simulink model "ex05_target_fio2_track_object_demo"  (Simulink 7.3)
settings: Solver=FixedStepDiscrete  SolverMode=SingleTasking  StartTime=0.0  StopTime=1  RelTol=1e-3
PreLoadFcn:
  | waijung.modelPreload; % Required for working with Waijung Blockset. Do not remove.
undefined symbols (not defined in the file): A1, A2, A7, B10, B11, B12, C1, C2, C3, C4, C5, Custom, G14, H2, H3, H6, H7, Link, LQFP176, ST, STM32F417IG, system_stm32f4xx
libraries: simulink x11, stm32f4_i2c_lib x8, viptextngfix x2, stm32f4_tim_lib x2, waijung_addon_module x2, waijung_webserver x2, dspsigattribs x1, waijung_image_sensor_lib x1, stm32f4_fsmc_lib x1, stm32f4_rcc_lib x1, stm32f4_device_config_lib x1, waijung_socket_lib x1
(part 1 of 2)
CloseFcn:
  | waijung.modelClose; % Required for working with Waijung Blockset. Do not remove.
settings Model: Creator=Krisada  LastModifiedBy=Krisada
settings OptimizationCC: EnhancedBackFolding=on  OptimizeModelRefInitCode=on  LifeSpan=1
settings HardwareCC: ProdEndianess=LittleEndian  ProdHWDeviceType=ARM Compatible->Cortex - M4  TargetEndianess=LittleEndian  TargetHWDeviceType=ARM Compatible->Cortex - M4
settings RTWCC: SystemTargetFile=stm32f4.tlc  GenerateMakefile=off  TemplateMakefile=ert_default_tmf  Description=STM32F4 Target  ProcessScript=stm32f4_make_rtw_hook
settings CodeAppCC: IgnoreCustomStorageClasses=off
settings STFCustomTargetCC: ModelReferenceCompliant=off  CombineOutputUpdateFcns=on  ERTCustomFileBanners=on  SupportContinuousTime=off  SupportNonInlinedSFcns=off  SystemTargetFile=stm32f4.tlc
settings ERTTargetCC: MultiwordLength=2048  ModelReferenceCompliant=off  ParMdlRefBuildCompliant=off  CompOptLevelCompliant=off  ERTFirstTimeCompliant=off  ModelStepFunctionPrototypeControlCompliant=off  CPPClassGenCompliant=off  ExtModeMexFile=noextcomm  InlinedParameterPlacement=NonHierarchical  ERTSrcFileBannerTemplate=stm32f4_code_template.cgt  ERTHdrFileBannerTemplate=stm32f4_code_template.cgt  ERTDataSrcFileTemplate=stm32f4_code_template.cgt  ERTDataHdrFileTemplate=stm32f4_code_template.cgt  ERTCustomFileTemplate=stm32f4_file_process.tlc

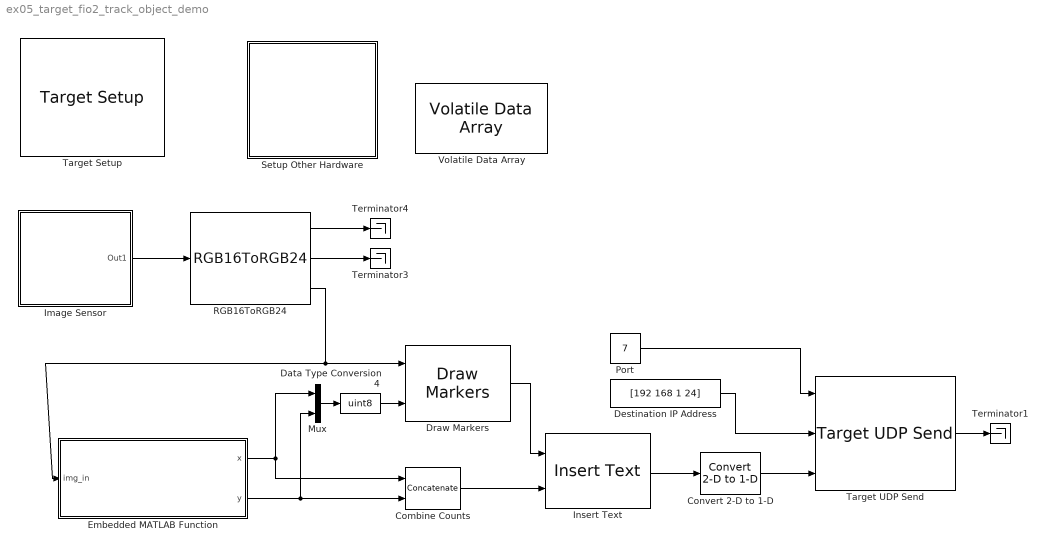
== system ex05_target_fio2_track_object_demo ==
  Combine Counts : Concatenate  Mode=Multidimensional array  ConcatenateDimension=2
  Convert 2-D to 1-D : dspsigattribs/Convert 2-D to 1-D  SystemSampleTime=-1
  Data Type Conversion4 : DataTypeConversion  OutDataTypeMode=uint8  OutDataType=fixdt(1, 16)  OutScaling=2^0  OutDataTypeStr=uint8
  Destination IP Address : Constant  Value=[192 168 1 24]  OutDataTypeMode=uint8  OutDataType=fixdt(1, 16)  OutScaling=2^0  OutDataTypeStr=uint8
  Draw Markers : viptextngfix/Draw Markers  DialogController=vipDDGCreate  DialogControllerArgs=DataTag0  shape=Square  size=5  fill=on  fillClrSource=Specify via dialog  display=White  intensity=200  color=1.5  opacity=0.6  viewport=Entire image  antialiasing=off  inType=Obsolete  imagePorts=One multidimensional signal  prodOutputMode=Binary point scaling  prodOutputWordLength=32  prodOutputFracLength=14  memoryMode=Specify word length  memoryWordLength=16  memoryFracLength=14  roundingMode=Floor  overflowMode=off
  Embedded MATLAB Function : Stateflow chart
  Image Sensor : Subsystem
  Insert Text : viptextngfix/Insert Text  DialogController=vipDDGCreate  DialogControllerArgs=DataTag1  inputType=Obsolete  theText='x: %3.2f, y: %3.2f'  fontFace=LucidaSansRegular  dummyVar1=0  blockFontSize=12  antiAliased=on  getTextLocFrom=Specify via dialog  textLoc=[5 5]  getTextColorFrom=Specify via dialog  textColor=[255 0 0]  getTextIntensityFrom=Specify via dialog  textIntensity=0  getTextOpacityFrom=Specify via dialog  textOpacity=1.0  dummyVar2=0  dummyVar3=0  dummyVar4=0  imagePorts=One multidimensional signal  isInputTransposed=off
  Mux : Mux  Inputs=2
  Port : Constant  Value=7  OutDataTypeMode=uint16  OutDataType=fixdt(1, 16)  OutScaling=2^0  OutDataTypeStr=uint16
  RGB16ToRGB24 : waijung_image_sensor_lib/RGB16ToRGB24  conf=RGB16ToRGB24  column=120  row=160  inputalignment=RGB  outputalignment=BGR  colorseparate=on  simparams=[0 160 0 1]  portpinstr=0  sampletime=-1  blockid=RGB16ToRGB24  inputporttype=[5]  inputportwidth=[19200]  inputportlabel={'Input'}  outputporttype="[3  3 3]"  outputportwidth=[120 120 120]  outputportlabel={'B','G','R'}  compat=0  optionstring="[\"BGR\",\"Param1\"]"
  Setup Other Hardware : Subsystem
  Target Setup : stm32f4_device_config_lib/Target Setup  Priority=100  compiler=GNU ARM  previous_compiler=GNU ARM  mcu=STM32F417IG (LQFP176)  mcustr=STM32F417IG  clockconfig=Custom (system_stm32f4xx.c)  system_stm32f4xx_c_path=F:\trunk\targets\stm32f4_target\stm32f4\utils\STM32F4xx_AN3988_V1.1.0  showmemoryconfiguration=on  stacksize=0x2000  heapsize=0x2000  enableautocompiledownload=on  fullchiperase=off  programmerinterface=ST-Link  editctrlstr=on  compilercontrolstr=$(patsubst %, -I%, .) -mcpu=cortex-m4 -mthumb -mthumb-interwork -mfloat-abi=hard -mfpu=fpv4-sp-d16 -ffast-math -Wall -Wextra -Ofast  assemblercontrolstr=$(patsubst %, -I%, .) -mcpu=cortex-m4 -mthumb -mthumb-interwork -mfloat-abi=hard -mfpu=fpv4-sp-d16 -ffast-math -Wall -Wextra -Ofast -Wa,-amhls=$(<:.s=.lst) -D__STACK_SIZE=$(STACK_SIZE) -D__HEAP_SIZE=$(HEAP_SIZE)  linkercontrolstr=-T$(LD_SCRIPT) -g -Wl,-Map=$(MAP),--cref,--no-warn-mismatch -mcpu=cortex-m4 -mthumb -mthumb-interwork -mfloat-abi=hard -mfpu=fpv4-sp-d16 -specs=nosys.specs  runafterdownload=on  execprofile=None  profileruart=4  profilerbaud=500000  profilertxpin=D8  profilerinitstr=0.01,168000000,1680000,500000,0  manualsetsampletime=off  sampletime=0.01  blockid=TargetSetup  systickreloadvalue=1680000  hseval=8000000  lastprofileruart=4  hclk=168000000  flashorigin=0x8000000  flashlength=1024k  ramorigin=0x64000000  ramlength=0x80000  useextram=on
  Target UDP Send : waijung_socket_lib/Target UDP Send  conf=TargetSend  protocol=UDP  variableipport=on  port=7  address=192.168.1.24  echo=off  transfer=Non-blocking  timeout=5  datasource=VectorStream  streamsource=ExtRAM  streamsize=512  datatype=uint8  datacount=19200  porttype_double=0  porttype_single=0  porttype_int8=0  porttype_uint8=0  porttype_int16=0  porttype_uint16=0  porttype_int32=0  porttype_uint32=1  portpinstr=0  sampletime=-1  blockid=TargetUDPSend  inputporttype=[5,3,3]  inputportwidth=[1,4,19200]  inputportlabel={'Port','IP','Data(1:19200)'}  outputporttype=[7]  outputportwidth=[]  outputportlabel={'Status'}  compat=0  optionstring="[\"UDP\",\"7\",\"192\",\"168\",\"1\",\"24\",\"Non-blocking\",\"VectorStream\",\"uint8_t\",\"19200\",\"Send\",\"off\",\"on\",\"\",\"\",\"\",\"\",\"\",\"512\"]"  options=[7,2,0,5000,0]
  Terminator1 : Terminator
  Terminator3 : Terminator
  Terminator4 : Terminator
  Volatile Data Array : waijung_addon_module/Data Storage/Volatile Data Array  conf=Setup  specificaddress=off  storagename=ExtRAM  memoryaddress=hex2dec('64000000')  storagetype=uint16  datasize=160*120  varname=VolatileDataArray_ExtRAM  datatype=double  datacount=0  portpinstr=0  sampletime=inf  blockid=VolatileDataArray  inputporttype=[]  inputportwidth=[]  inputportlabel={}  outputporttype=[]  outputportwidth=[]  outputportlabel={}  compat=0  optionstring="[\"off\",\"?\",\"ExtRAM\",\"uint16\",\"19200\",\"VolatileDataArray_ExtRAM\",\"uint16_t\",\"Param1\"]"
  wires:
  Image Sensor/1(Out1) -> RGB16ToRGB24/1
  RGB16ToRGB24/2 -> Terminator3/1
  RGB16ToRGB24/1 -> Terminator4/1
  Mux/1 -> Data Type Conversion4/1
  Data Type Conversion4/1 -> Draw Markers/2
  Draw Markers/1 -> Insert Text/1
  Combine Counts/1 -> Insert Text/2
  Embedded MATLAB Function/1(x) -> Mux/1, Combine Counts/1
  Embedded MATLAB Function/2(y) -> Mux/2, Combine Counts/2
  Insert Text/1 -> Convert 2-D to 1-D/1
  Destination IP Address/1 -> Target UDP Send/2
  Port/1 -> Target UDP Send/1
  Target UDP Send/1 -> Terminator1/1
  Convert 2-D to 1-D/1 -> Target UDP Send/3
  RGB16ToRGB24/3 -> Embedded MATLAB Function/1(img_in), Draw Markers/1

== system ex05_target_fio2_track_object_demo/Image Sensor ==
  Camera OV1 : Subsystem  mask{camera=OV7670, storagename=ExtRAM, xclkfreq=8MHz(MCO), imgsize=120 x 160, module=1, slvaddr=hex2dec('42'), sampletime=0.1}
      mask prompts: storagename "Output buffer"; xclkfreq "XCLK input frequency"; imgsize "Image size"; module "I2C Module"; slvaddr "I2C Slave address"; sampletime "Sample time (sec)"
      mask init:
      | waijung_image_sensor_callback('init');
      mask StyleString: popup(OV7670),popup(ExtRAM|ExtRAM),popup(8MHz(MCO)|24MHz),popup(120 x 160|240 x 320|480 x 640),popup(1|2|3),edit,edit
      mask CallbackString: waijung_image_sensor_callback('camera');|waijung_image_sensor_callback('storagename');|||waijung_image_sensor_callback('module');||
      mask Display: text(0.5, 0.5, '[OV7670]\nPort: I2C1','ver','middle','hor','center');port_label('output', 1,'READY');
  Constant2 : Constant  Value=0  OutDataTypeMode=uint32  OutDataType=fixdt(1, 16)  OutScaling=2^0  OutDataTypeStr=uint32  SampleTime=0.1
  Terminator : Terminator
  Volatile Data Array Read : waijung_addon_module/Data Storage/Volatile Data Array Read  conf=Read  specificaddress=off  storagename=ExtRAM  memoryaddress=hex2dec('64000000')  storagetype=uint8  datasize=120*160*3  varname=VolatileDataArray_ExtRAM  datatype=uint8  datacount=128  variablesize=off  portpinstr=0  sampletime=inf  blockid=ImageSensorVolatileDataArrayRead  inputporttype=[7]  inputportwidth=[1]  inputportlabel={'Offset'}  outputporttype=[3]  outputportwidth=[128]  outputportlabel={'Data(128)'}  compat=0  optionstring="[\"ExtRAM\",\"uint16\",\"19200\",\"VolatileDataArray_ExtRAM\",\"uint16_t\",\"uint16\",\"uint16_t\",\"19200\",\"Param1\"]"
  Out1 : Outport
  wires:
  Constant2/1 -> Volatile Data Array Read/1
  Camera OV1/1(Data) -> Terminator/1
  Volatile Data Array Read/1 -> Out1/1

== system ex05_target_fio2_track_object_demo/Setup Other Hardware ==
  Ethernet Application Setup : waijung_webserver/Ethernet Application Setup  conf=Setup  ipaddress=192.168.1.31  netmask=255.255.255.0  gateway=192.168.1.1  macaddress=02-00-00-00-00-00  dhcp=off  timerscaler=100  portpinstr=0  sampletime=0.0001  blockid=SetupOtherHardwareEthernetApplicationSetup  inputporttype=[]  inputportwidth=[]  inputportlabel={}  outputporttype=[]  outputportwidth=[]  outputportlabel={}  compat=0  optionstring="[\"Dummy\",\"192\",\"168\",\"1\",\"31\",\"255\",\"255\",\"255\",\"0\",\"192\",\"168\",\"1\",\"1\",\"02\",\"00\",\"00\",\"00\",\"00\",\"00\",\"off\",\"100\"]"
  Ethernet Link Setup1 : waijung_webserver/Ethernet Link Setup  conf=Setup  interfacepin=Profile #2  wj_interfacetype=MII  pin_mdio=A2  pin_mdc=C1  pin_pps=Not used  pin_crs=H2  pin_col=H3  pin_dv=A7  pin_rxclk=A1  pin_rxer=B10  pin_rxd0=C4  pin_rxd1=C5  pin_rxd2=H6  pin_rxd3=H7  pin_txclk=C3  pin_txen=B11  pin_txd0=B12  pin_txd1=G14  pin_txd2=C2  pin_txd3=E2  portpinstr=H2,A1,A2,H3,A7,H6,H7,E2,B10,B11,B12,G14,C1,C2,C3,C4,C5  sampletime=inf  blockid=SetupOtherHardwareEthernetLinkSetup1  inputporttype=[]  inputportwidth=[]  inputportlabel={}  outputporttype=[]  outputportwidth=[]  outputportlabel={}  compat=0  optionstring="[\"xxx\",\"on\",\"on\",\"on\",\"off\",\"on\",\"off\",\"on\",\"on\",\"off\",\"on\",\"on\",\"on\",\"on\",\"on\",\"on\",\"on\",\"off\",\"on\",\"on\",\"on\",\"on\",\"on\",\"on\",\"on\",\"on\",\"on\",\"on\",\"H\",\"2\",\"A\",\"1\",\"A\",\"2\",\"H\",\"3\",\"A\",\"7\",\"H\",\"6\",\"H\",\"7\",\"N\",\"ot used\",\"E\",\"2\",\"B\",\"10\",\"B\",\"11\",\"B\",\"12\",\"G\",\"14\",\"C\",\"1\",\"C\",\"2\",\"C\",\"3\",\"C\",\"4\",\"C\",\"5\",\"MII\"]"
  FSMC_SRAM Setup : stm32f4_fsmc_lib/FSMC_SRAM Setup  conf=RamSetup  useextmem=on  extmemaddress=hex2dec('64000000')  extramsize=hex2dec('80000')  datasource=0x64000000  sampletime=inf  sampletimestr=0  blockid=SetupOtherHardwareFSMC_SRAMSetup  inputarray=[]  inputlabelarray={}  outputarray=[]  outputlabelarray={}  compat=0  confstr="[\"on\"]"
  I2C Master Setup : S-Function  FunctionName=stm32f4_i2c  Parameters=configuration,module,transfer,clkspeed,timeout,sdapin,sclpin,writecount,readcount,inputtypearray,outputtypearray,confstr,sampletime,sampletimestr,blockid  EnableBusSupport=off  mask(stm32f4_i2c){configuration=Setup, module=1, lastmodule=1, transfer=Blocking, dutycycle=TLow/THigh = 2, clkspeed=100, timeout=25, writecount=0, readcount=0, sdapin=B7, sclpin=B6, waitwritetime=0, inputtypearray=[0], outputtypearray=[0], confstr=["B","7","B","6","1","1","6","0","I2C_DutyCycle_2","0","off"], sampletime=-1, sampletimestr=0, blockid=SetupOtherHardwareI2CMasterSetup}
      mask prompts: module "I2C Module"; lastmodule "Last module"; transfer "Transfer mode"; dutycycle "Duty cycle in fast mode"; clkspeed "Clock speed (kHz)"; timeout "Timeout (ms)"; writecount "Bytes write count"; readcount "Bytes read count"; sdapin "SDA pin"; sclpin "SCL pin"; waitwritetime "Wait write time (ms), default is 0"; inputtypearray "Input type array"; outputtypearray "Output type array"; confstr "Configuration string"; sampletime "Sample time (sec)"; sampletimestr "Compiled sample time (sec) in string"
      mask init:
      | stm32f4_i2c_callback('init');
      mask Help: web(fullfile(waijungdocroot,'stm32f4_i2c_setup.htm'), '-browser')
      mask StyleString: popup(Setup|Transaction),popup(1|2|3),edit,popup(Blocking|Non-blocking),popup(TLow/THigh = 16/9|TLow/THigh = 2),edit,edit,edit,edit,popup(Not used|B7|B9),popup(Not used|B6|B8),edit,edit,edit,edit,edit,edit,edit
      mask CallbackString: stm32f4_i2c_callback('configuration');|stm32f4_i2c_callback('module');|||stm32f4_i2c_callback('dutycycle');|||stm32f4_i2c_callback('writecount');|stm32f4_i2c_callback('readcount');|stm32f4_i2c_callback('sdapin');|stm32f4_i2c_callback('sclpin');||||stm32f4_i2c_callback('confstr');|stm32f4_i2c_callback('sampletime');|stm32f4_i2c_callback('sampletimestr');|stm32f4_i2c_callback('blockid');
      mask Display: text(0.5, 0.5, 'Module: I2C1\nClock: 100kHz\nSDA/SCL Pin: B7/B6','ver','middle','hor','center');
  MCO : stm32f4_rcc_lib/MCO  conf=MCO  module=1  source=HSE  div=Div_1  sampletime=inf  sampletimestr=0  blockid=SetupOtherHardwareMCO  inputarray=[]  inputlabelarray={}  outputarray=[]  outputlabelarray={}  compat=0  confstr="[\"1\",\"HSE\",\"Div_1\"]"

== system ex05_target_fio2_track_object_demo/Image Sensor/Camera OV1 ==
  Capture_ : Subsystem  TreatAsAtomicUnit=on
  Init_ : Subsystem
  Logical Operator : Logic  Operator=NOT  AllPortsSameDT=off  OutDataTypeMode=boolean  LogicDataType=fixdt(0, 8)  OutDataTypeStr=boolean
  Memory : Memory  InheritSampleTime=on
  Rate Transition : RateTransition  OutPortSampleTime=sampletime
  Data : Outport  OutDataType=fixdt(1, 16)  OutScaling=2^0
  wires:
  Rate Transition/1 -> Capture_/Enable
  Logical Operator/1 -> Init_/Enable
  Memory/1 -> Rate Transition/1, Logical Operator/1
  Init_/1(Out1) -> Memory/1
  Capture_/1(SUCCESS) -> Data/1

== system ex05_target_fio2_track_object_demo/Image Sensor/Camera OV1/Capture_ ==
  Enable : EnablePort
  Compare To Zero : simulink/Logic and Bit Operations/Compare To Zero  SystemSampleTime=-1  relop===  LogicOutDataTypeMode=uint8  ZeroCross=off
  DCMI Capture : S-Function  FunctionName=stm32f4_dcmi  Parameters=conf,inputporttype,inputportwidth,outputporttype,outputportwidth,optionstring,sampletime,blockid  EnableBusSupport=off  mask(stm32f4_dcmi){conf=DCMI, capturemode=SnapShot, synchronizemode=Hardware, pclkpolarity=Falling, vspolarity=High, hspolarity=High, capturerate=All, capturesize=120*160*2, storagename=<Manual Configure>, varname=VolatileDataArray_ExtRAM, storagetype=uint16, storagesize=120*160, remap=Profile #2, sampletime=inf, blockid=ImageSensorCameraOV1Capture_DCMICapture, inputporttype=[], inputportwidth=[], inputportlabel={}, outputporttype=[7], outputportwidth=[], outputportlabel={'Status'}, compat=0, optionstring=["DCMI","SnapShot","Hardware","Falling","High","High","All","0","HalfWord","9600","0","0","VolatileDataArray_ExtRAM"," "," "," ","1","0","0","0","0","0","0","1","1","A","6","I","5","H","8","H","9","H","10","H","11","H","12","H","14","I","4","I","6","I","7"], portpinstr=A6,I5,H8,H9,H10,H11,H12,H14,I4,I6,I7}
      mask prompts: conf "Configuration"; capturemode "Capture mode"; synchronizemode "Synchronization Mode"; pclkpolarity "Pixel clock polarity"; vspolarity "Vertical synchronization polarity"; hspolarity "Horizontal synchronization polarity"; capturerate "Capture rate"; capturesize "Capture data size (Bytes)"; storagename "Output buffer"; varname "Output buffer var name"; storagetype "Output buffer var type"; storagesize "Output buffer size (Total bytes must be equal to, or greater than DMA Transfer size)"; remap "Remap DCMI pins"; sampletime "Sample time (sec)"; inputporttype "Input port"; inputportwidth "Input Port Width"; inputportlabel "Input port label"; outputporttype "Output port"; outputportwidth "Output Port Width"; outputportlabel "Output port label"; compat "Compatibility (Reserved for future use)"; optionstring "Configuration String"; portpinstr "Port Pin String"
      mask help:
      | Synchronize mode:
      |  - Hardware: Hardware synchronization data capture is synchronized with the HSYNC/VSYNC signals.
      |  - Embedded: Embedded synchronization data capture is synchronized with synchronization codes embedded in the data flow.
      | Pixel clock polarity:
      |  - Falling: Pixel clock active on Falling edge.
      |  - Rising: Pixel clock active on Rising edge.
      | Vertical, Horizontal sychronization polarity:
      |  - Low: vertical synchronization active Low.
      |  - High: Vertical synchronization active High.
      | Capture rate:
      |  - All: All frames are captured.
      |  - 1of2: Every alternate frame captured.
      |  - 1of4: On frame in 4 frames captured.
      | Pins Profile:
      | Set of configuration pins for: PIXCLK, VSYNC, HSYNC, D0, D1, .., D7 corresponding.
      |  - Profile #1: PA6, PB7, PA4, PC6, PC7,  PE0,  PE1,  PE4,  PB6, PE5, PE6
      |  - Profile #2: PA6, PI5, PH8, PH9, PH10, PH11, PH12, PH14, PI4, PI6, PI7
      mask init:
      | stm32f4_dcmi_callback('init');
      mask Help: web(fullfile(waijungdocroot,'stm32f4_dcmi.htm'), '-browser')
      mask StyleString: popup(DCMI),popup(Continuous|SnapShot),popup(Hardware|Embedded),popup(Falling|Rising),popup(High|Low),popup(High|Low),popup(All|1of2|1of4),edit,popup(<Manual Configure>),edit,popup(double|single|int8|uint8|int16|uint16|int32|uint32),edit,popup(Profile #1|Profile #2),edit,edit,edit,edit,edit,edit,edit,edit,edit,edit,edit
      mask CallbackString: stm32f4_dcmi_callback('conf');||||||||stm32f4_dcmi_callback('storagename');|||stm32f4_dcmi_callback('storagesize');|stm32f4_dcmi_callback('remap');|stm32f4_dcmi_callback('sampletime');|stm32f4_dcmi_callback('blockid');|||||||||
      mask Display: text(0.05, 0.5, 'Size: 38400\nPins: Profile #2\nTs (sec): 0','ver','middle','hor','left'); port_label('output', 1,'Status');
  SUCCESS : Outport  OutDataType=fixdt(1, 16)  OutScaling=2^0
  wires:
  DCMI Capture/1 -> Compare To Zero/1
  Compare To Zero/1 -> SUCCESS/1

== system ex05_target_fio2_track_object_demo/Image Sensor/Camera OV1/Init_ ==
  Enable : EnablePort
  While Iterator_ : Subsystem  TreatAsAtomicUnit=on
  Out1 : Outport
  wires:
  While Iterator_/1(Ready) -> Out1/1

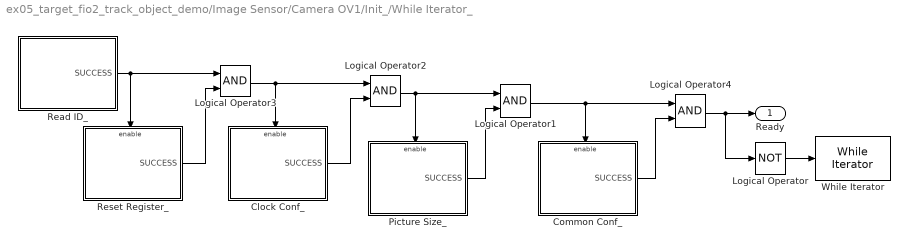
== system ex05_target_fio2_track_object_demo/Image Sensor/Camera OV1/Init_/While Iterator_ ==
  Clock Conf_ : Subsystem
  Common Conf_ : Subsystem
  Logical Operator : Logic  Operator=NOT  AllPortsSameDT=off  OutDataTypeMode=boolean  LogicDataType=fixdt(0, 8)  OutDataTypeStr=boolean
  Logical Operator{1..4} (4 alike) : Logic  AllPortsSameDT=off  OutDataTypeMode=boolean  LogicDataType=fixdt(0, 8)  OutDataTypeStr=boolean
  Picture Size_ : Subsystem
  Read ID_ : Subsystem
  Reset Register_ : Subsystem
  While Iterator : WhileIterator  MaxIters=-1  WhileBlockType=do-while
  Ready : Outport  OutDataType=fixdt(1, 16)  OutScaling=2^0
  wires:
  Common Conf_/1(SUCCESS) -> Logical Operator4/2
  Logical Operator4/1 -> Ready/1, Logical Operator/1
  Logical Operator2/1 -> Picture Size_/Enable, Logical Operator1/1
  Clock Conf_/1(SUCCESS) -> Logical Operator2/2
  Reset Register_/1(SUCCESS) -> Logical Operator3/2
  Logical Operator/1 -> While Iterator/1
  Logical Operator1/1 -> Logical Operator4/1, Common Conf_/Enable
  Picture Size_/1(SUCCESS) -> Logical Operator1/2
  Read ID_/1(SUCCESS) -> Logical Operator3/1, Reset Register_/Enable
  Logical Operator3/1 -> Logical Operator2/1, Clock Conf_/Enable

== system ex05_target_fio2_track_object_demo/Image Sensor/Camera OV1/Init_/While Iterator_/Clock Conf_ ==
  Enable : EnablePort
  Logical Operator : Logic  Operator=NOT  AllPortsSameDT=off  OutDataTypeMode=boolean  LogicDataType=fixdt(0, 8)  OutDataTypeStr=boolean
  Memory : Memory  InheritSampleTime=on
  Subsystem : Subsystem
  SUCCESS : Outport  OutDataType=fixdt(1, 16)  OutScaling=2^0
  wires:
  Subsystem/1(Out1) -> SUCCESS/1, Memory/1
  Logical Operator/1 -> Subsystem/Enable
  Memory/1 -> Logical Operator/1

== system ex05_target_fio2_track_object_demo/Image Sensor/Camera OV1/Init_/While Iterator_/Common Conf_ ==
  Enable : EnablePort
  Logical Operator : Logic  Operator=NOT  AllPortsSameDT=off  OutDataTypeMode=boolean  LogicDataType=fixdt(0, 8)  OutDataTypeStr=boolean
  Memory : Memory  InheritSampleTime=on
  Subsystem : Subsystem
  SUCCESS : Outport  OutDataType=fixdt(1, 16)  OutScaling=2^0
  wires:
  Subsystem/1(Out1) -> SUCCESS/1, Memory/1
  Logical Operator/1 -> Subsystem/Enable
  Memory/1 -> Logical Operator/1

== system ex05_target_fio2_track_object_demo/Image Sensor/Camera OV1/Init_/While Iterator_/Picture Size_ ==
  Enable : EnablePort
  Logical Operator : Logic  Operator=NOT  AllPortsSameDT=off  OutDataTypeMode=boolean  LogicDataType=fixdt(0, 8)  OutDataTypeStr=boolean
  Memory : Memory  InheritSampleTime=on
  Subsystem : Subsystem
  SUCCESS : Outport  OutDataType=fixdt(1, 16)  OutScaling=2^0
  wires:
  Memory/1 -> Logical Operator/1
  Logical Operator/1 -> Subsystem/Enable
  Subsystem/1(Out1) -> Memory/1, SUCCESS/1

== system ex05_target_fio2_track_object_demo/Image Sensor/Camera OV1/Init_/While Iterator_/Read ID_ ==
  Logical Operator : Logic  Operator=NOT  AllPortsSameDT=off  OutDataTypeMode=boolean  LogicDataType=fixdt(0, 8)  OutDataTypeStr=boolean
  Memory : Memory  InheritSampleTime=on
  Subsystem_ : Subsystem
  SUCCESS : Outport  OutDataType=fixdt(1, 16)  OutScaling=2^0
  wires:
  Memory/1 -> Logical Operator/1
  Logical Operator/1 -> Subsystem_/Enable
  Subsystem_/1(Out1) -> Memory/1, SUCCESS/1

== system ex05_target_fio2_track_object_demo/Image Sensor/Camera OV1/Init_/While Iterator_/Reset Register_ ==
  Enable : EnablePort
  Logical Operator : Logic  Operator=NOT  AllPortsSameDT=off  OutDataTypeMode=boolean  LogicDataType=fixdt(0, 8)  OutDataTypeStr=boolean
  Memory : Memory  InheritSampleTime=on
  Subsystem : Subsystem
  SUCCESS : Outport  OutDataType=fixdt(1, 16)  OutScaling=2^0
  wires:
  Subsystem/1(Out1) -> SUCCESS/1, Memory/1
  Logical Operator/1 -> Subsystem/Enable
  Memory/1 -> Logical Operator/1

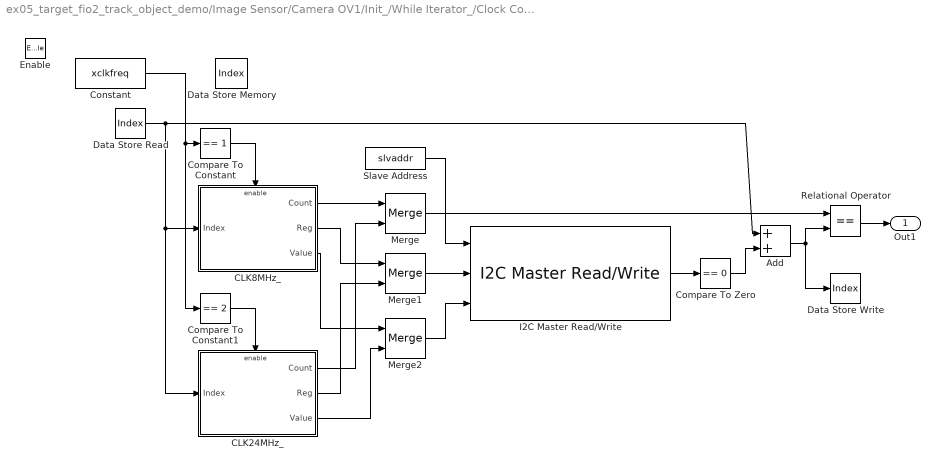
== system ex05_target_fio2_track_object_demo/Image Sensor/Camera OV1/Init_/While Iterator_/Clock Conf_/Subsystem ==
  Enable : EnablePort
  Add : Sum  OutDataType=fixdt(1, 16)  OutScaling=2^-10
  CLK24MHz_ : Subsystem  TreatAsAtomicUnit=on
  CLK8MHz_ : Subsystem  TreatAsAtomicUnit=on
  Compare To Constant : simulink/Logic and Bit Operations/Compare To Constant  SystemSampleTime=-1  relop===  const=1  LogicOutDataTypeMode=boolean  ZeroCross=off
  Compare To Constant1 : simulink/Logic and Bit Operations/Compare To Constant  SystemSampleTime=-1  relop===  const=2  LogicOutDataTypeMode=boolean  ZeroCross=off
  Compare To Zero : simulink/Logic and Bit Operations/Compare To Zero  SystemSampleTime=-1  relop===  LogicOutDataTypeMode=uint8  ZeroCross=off
  Constant : Constant  Value=xclkfreq  OutDataType=fixdt(1, 16)  OutScaling=2^0
  Data Store Memory : DataStoreMemory  DataStoreName=Index  ReadBeforeWriteMsg=warning  WriteAfterWriteMsg=warning  WriteAfterReadMsg=warning  DataType=uint8  OutDataType=fixdt(1, 16)  OutScaling=2^0  OutDataTypeStr=uint8
  Data Store Read : DataStoreRead  DataStoreName=Index  SampleTime=-1
  Data Store Write : DataStoreWrite  DataStoreName=Index  SampleTime=-1
  I2C Master Read/Write : stm32f4_i2c_lib/I2C Master Read//Write  configuration=Transaction  module=1  lastmodule=3  transfer=Blocking  dutycycle=TLow/THigh = 2  clkspeed=400  timeout=25  writecount=2  readcount=0  sdapin=C9  sclpin=A8  waitwritetime=5  forcestop=off  inputtypearray=[3 3 3 3]  outputtypearray=[1 3]  confstr="[\"C\",\"9\",\"A\",\"8\",\"1\",\"1\",\"6\",\"0\",\"I2C_DutyCycle_2\",\"5\",\"off\"]"  sampletime=-1  sampletimestr=0  blockid=ImageSensorCameraOV1Init_WhileIterator_ClockConf_SubsystemI2CMasterReadWrite
  Merge : Merge
  Merge1 : Merge
  Merge2 : Merge
  Relational Operator : RelationalOperator  Operator===  LogicOutDataTypeMode=boolean  LogicDataType=fixdt(0, 8)  OutDataTypeStr=boolean
  Slave Address : Constant  Value=slvaddr  OutDataTypeMode=uint8  OutDataType=fixdt(1, 16)  OutScaling=2^0  OutDataTypeStr=uint8
  Out1 : Outport
  wires:
  Merge2/1 -> I2C Master Read/Write/3
  Merge1/1 -> I2C Master Read/Write/2
  Merge/1 -> Relational Operator/1
  Constant/1 -> Compare To Constant1/1, Compare To Constant/1
  CLK24MHz_/3(Value) -> Merge2/2
  CLK24MHz_/2(Reg) -> Merge1/2
  CLK24MHz_/1(Count) -> Merge/2
  CLK8MHz_/3(Value) -> Merge2/1
  CLK8MHz_/2(Reg) -> Merge1/1
  CLK8MHz_/1(Count) -> Merge/1
  Compare To Constant1/1 -> CLK24MHz_/Enable
  Compare To Constant/1 -> CLK8MHz_/Enable
  Slave Address/1 -> I2C Master Read/Write/1
  Data Store Read/1 -> CLK24MHz_/1(Index), CLK8MHz_/1(Index), Add/1
  I2C Master Read/Write/1 -> Compare To Zero/1
  Compare To Zero/1 -> Add/2
  Add/1 -> Relational Operator/2, Data Store Write/1
  Relational Operator/1 -> Out1/1

== system ex05_target_fio2_track_object_demo/Image Sensor/Camera OV1/Init_/While Iterator_/Common Conf_/Subsystem ==
  Enable : EnablePort
  Add : Sum  OutDataType=fixdt(1, 16)  OutScaling=2^-10
  Compare To Zero : simulink/Logic and Bit Operations/Compare To Zero  SystemSampleTime=-1  relop===  LogicOutDataTypeMode=uint8  ZeroCross=off
  Data Store Memory : DataStoreMemory  DataStoreName=Index  ReadBeforeWriteMsg=warning  WriteAfterWriteMsg=warning  WriteAfterReadMsg=warning  DataType=uint8  OutDataType=fixdt(1, 16)  OutScaling=2^0  OutDataTypeStr=uint8
  Data Store Read : DataStoreRead  DataStoreName=Index  SampleTime=-1
  Data Store Write : DataStoreWrite  DataStoreName=Index  SampleTime=-1
  I2C Master Read/Write : stm32f4_i2c_lib/I2C Master Read//Write  configuration=Transaction  module=1  lastmodule=3  transfer=Blocking  dutycycle=TLow/THigh = 2  clkspeed=400  timeout=25  writecount=2  readcount=0  sdapin=C9  sclpin=A8  waitwritetime=5  forcestop=off  inputtypearray=[3 3 3 3]  outputtypearray=[1 3]  confstr="[\"C\",\"9\",\"A\",\"8\",\"1\",\"1\",\"6\",\"0\",\"I2C_DutyCycle_2\",\"5\",\"off\"]"  sampletime=-1  sampletimestr=0  blockid=ImageSensorCameraOV1Init_WhileIterator_CommonConf_SubsystemI2CMasterReadWrite
  Register List : Subsystem  mask{register=uint8([122,123,124,125,126,127,128,129,130,131,132,133,134,135,136,137,19,21,0,16,13,20,165,171,36,37,38,159,160,161,166,167,168,169,170,19,14,15,22,30,33,34,41,51,53,55,56,57,60,77,78,105,116,141,142,143,144,145,146,150,154,176,177,178,179,184,67,68,69,70,71,72,89,90,91,92,93,94,100,101,102,148,149,108,109,110,111,106,1,2,19,21,79,80,81,82,83,84,85,86,87,88,65,63,117,118,76,119,75,201,65,86,52,59,164,150,157,158,9,59]), value=uint8([32,28,40,60,85,104,118,128,136,143,150,163,175,196,215,232,232,24,15,0,0,32,5,7,117,99,165,120,104,3,223,223,240,144,148,229,97,75,2,39,2,145,7,11,11,29,113,42,120,64,32,0,25,79,0,0,0,0,0,0,128,132,12,14,130,10,20,240,52,88,40,58,136,136,68,103,73,14,4,32,5,4,8,10,85,17,159,64,64,64,231,24,128,128,0,34,94,128,0,82,128,158,8,5,5,225,15,10,9,192,56,64,17,2,137,0,76,63,2,66])}
      mask prompts: register "Register Index"; value "Register Value"
      mask help:
      | Count:
      |  - Number of Register-Value pair.
      |  - Determine from lowest size, between Register and Value.
      | Reg:
      |  - Register index.
      | Value:
      |  - Data corresponding to specified register index.
  Relational Operator : RelationalOperator  Operator===  LogicOutDataTypeMode=boolean  LogicDataType=fixdt(0, 8)  OutDataTypeStr=boolean
  Slave Address : Constant  Value=slvaddr  OutDataTypeMode=uint8  OutDataType=fixdt(1, 16)  OutScaling=2^0  OutDataTypeStr=uint8
  Out1 : Outport
  wires:
  Slave Address/1 -> I2C Master Read/Write/1
  Data Store Read/1 -> Add/1, Register List/1(Index)
  I2C Master Read/Write/1 -> Compare To Zero/1
  Compare To Zero/1 -> Add/2
  Add/1 -> Relational Operator/2, Data Store Write/1
  Relational Operator/1 -> Out1/1
  Register List/2(Reg) -> I2C Master Read/Write/2
  Register List/3(Value) -> I2C Master Read/Write/3
  Register List/1(Count) -> Relational Operator/1

== system ex05_target_fio2_track_object_demo/Image Sensor/Camera OV1/Init_/While Iterator_/Picture Size_/Subsystem ==
  Enable : EnablePort
  Add : Sum  OutDataType=fixdt(1, 16)  OutScaling=2^-10
  Compare To Zero : simulink/Logic and Bit Operations/Compare To Zero  SystemSampleTime=-1  relop===  LogicOutDataTypeMode=uint8  ZeroCross=off
  Data Store Memory : DataStoreMemory  DataStoreName=Index  ReadBeforeWriteMsg=warning  WriteAfterWriteMsg=warning  WriteAfterReadMsg=warning  DataType=uint8  OutDataType=fixdt(1, 16)  OutScaling=2^0  OutDataTypeStr=uint8
  Data Store Read : DataStoreRead  DataStoreName=Index  SampleTime=-1
  Data Store Write : DataStoreWrite  DataStoreName=Index  SampleTime=-1
  I2C Master Read/Write : stm32f4_i2c_lib/I2C Master Read//Write  configuration=Transaction  module=1  lastmodule=3  transfer=Blocking  dutycycle=TLow/THigh = 2  clkspeed=400  timeout=25  writecount=2  readcount=0  sdapin=C9  sclpin=A8  waitwritetime=5  forcestop=off  inputtypearray=[3 3 3 3]  outputtypearray=[1 3]  confstr="[\"C\",\"9\",\"A\",\"8\",\"1\",\"1\",\"6\",\"0\",\"I2C_DutyCycle_2\",\"5\",\"off\"]"  sampletime=-1  sampletimestr=0  blockid=ImageSensorCameraOV1Init_WhileIterator_PictureSize_SubsystemI2CMasterReadWrite
  Relational Operator : RelationalOperator  Operator===  LogicOutDataTypeMode=boolean  LogicDataType=fixdt(0, 8)  OutDataTypeStr=boolean
  Slave Address : Constant  Value=slvaddr  OutDataTypeMode=uint8  OutDataType=fixdt(1, 16)  OutScaling=2^0  OutDataTypeStr=uint8
  Subsystem : Subsystem
  Out1 : Outport
  wires:
  Subsystem/1(Count) -> Relational Operator/1
  Subsystem/2(Reg) -> I2C Master Read/Write/2
  Subsystem/3(Value) -> I2C Master Read/Write/3
  Relational Operator/1 -> Out1/1
  Add/1 -> Data Store Write/1, Relational Operator/2
  Compare To Zero/1 -> Add/2
  I2C Master Read/Write/1 -> Compare To Zero/1
  Data Store Read/1 -> Subsystem/1(Index), Add/1
  Slave Address/1 -> I2C Master Read/Write/1

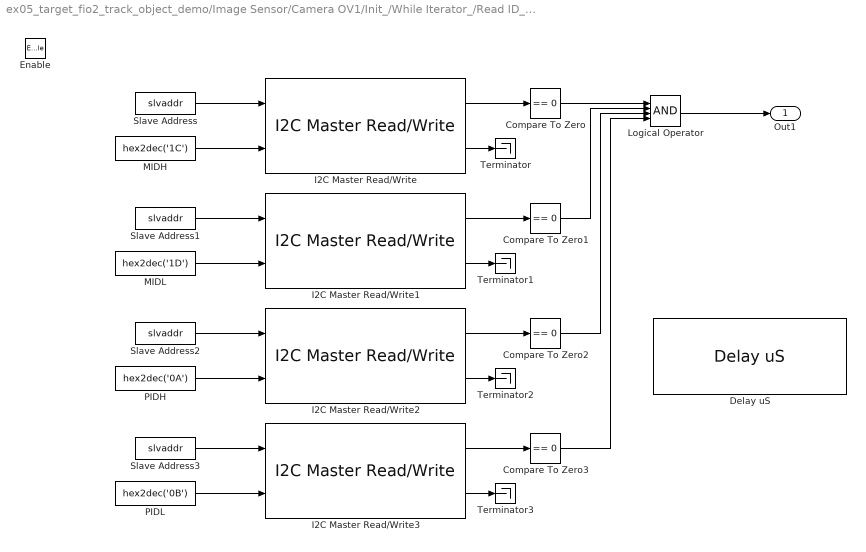
== system ex05_target_fio2_track_object_demo/Image Sensor/Camera OV1/Init_/While Iterator_/Read ID_/Subsystem_ ==
  Enable : EnablePort
  Compare To Zero{,1..3} (4 alike) : simulink/Logic and Bit Operations/Compare To Zero  SystemSampleTime=-1  relop===  LogicOutDataTypeMode=uint8  ZeroCross=off
  Delay uS : stm32f4_tim_lib/Delay uS  Priority=0  delaytime=300000  enableinput=off  enableoutput=off  inputtypearray=[0]  outputtypearray=[0]  sampletime=-1  sampletimestr=0  blockid=ImageSensorCameraOV1Init_WhileIterator_ReadID_Subsystem_DelayuS
  I2C Master Read/Write : stm32f4_i2c_lib/I2C Master Read//Write  configuration=Transaction  module=1  lastmodule=3  transfer=Blocking  dutycycle=TLow/THigh = 2  clkspeed=400  timeout=25  writecount=1  readcount=1  sdapin=C9  sclpin=A8  waitwritetime=0  forcestop=on  inputtypearray=[2 3 3]  outputtypearray=[2 3 3]  confstr="[\"C\",\"9\",\"A\",\"8\",\"1\",\"1\",\"6\",\"0\",\"I2C_DutyCycle_2\",\"0\",\"on\"]"  sampletime=-1  sampletimestr=0  blockid=ImageSensorCameraOV1Init_WhileIterator_ReadID_Subsystem_I2CMasterReadWrite
  I2C Master Read/Write1 : stm32f4_i2c_lib/I2C Master Read//Write  configuration=Transaction  module=1  lastmodule=3  transfer=Blocking  dutycycle=TLow/THigh = 2  clkspeed=400  timeout=25  writecount=1  readcount=1  sdapin=C9  sclpin=A8  waitwritetime=0  forcestop=on  inputtypearray=[2 3 3]  outputtypearray=[2 3 3]  confstr="[\"C\",\"9\",\"A\",\"8\",\"1\",\"1\",\"6\",\"0\",\"I2C_DutyCycle_2\",\"0\",\"on\"]"  sampletime=-1  sampletimestr=0  blockid=ImageSensorCameraOV1Init_WhileIterator_ReadID_Subsystem_I2CMasterReadWrite1
  I2C Master Read/Write2 : stm32f4_i2c_lib/I2C Master Read//Write  configuration=Transaction  module=1  lastmodule=3  transfer=Blocking  dutycycle=TLow/THigh = 2  clkspeed=400  timeout=25  writecount=1  readcount=1  sdapin=C9  sclpin=A8  waitwritetime=0  forcestop=on  inputtypearray=[2 3 3]  outputtypearray=[2 3 3]  confstr="[\"C\",\"9\",\"A\",\"8\",\"1\",\"1\",\"6\",\"0\",\"I2C_DutyCycle_2\",\"0\",\"on\"]"  sampletime=-1  sampletimestr=0  blockid=ImageSensorCameraOV1Init_WhileIterator_ReadID_Subsystem_I2CMasterReadWrite2
  I2C Master Read/Write3 : stm32f4_i2c_lib/I2C Master Read//Write  configuration=Transaction  module=1  lastmodule=3  transfer=Blocking  dutycycle=TLow/THigh = 2  clkspeed=400  timeout=25  writecount=1  readcount=1  sdapin=C9  sclpin=A8  waitwritetime=0  forcestop=on  inputtypearray=[2 3 3]  outputtypearray=[2 3 3]  confstr="[\"C\",\"9\",\"A\",\"8\",\"1\",\"1\",\"6\",\"0\",\"I2C_DutyCycle_2\",\"0\",\"on\"]"  sampletime=-1  sampletimestr=0  blockid=ImageSensorCameraOV1Init_WhileIterator_ReadID_Subsystem_I2CMasterReadWrite3
  Logical Operator : Logic  Inputs=4  AllPortsSameDT=off  OutDataTypeMode=boolean  LogicDataType=fixdt(0, 8)  OutDataTypeStr=boolean
  MIDH : Constant  Value=hex2dec('1C')  OutDataTypeMode=uint8  OutDataType=fixdt(1, 16)  OutScaling=2^0  OutDataTypeStr=uint8
  MIDL : Constant  Value=hex2dec('1D')  OutDataTypeMode=uint8  OutDataType=fixdt(1, 16)  OutScaling=2^0  OutDataTypeStr=uint8
  PIDH : Constant  Value=hex2dec('0A')  OutDataTypeMode=uint8  OutDataType=fixdt(1, 16)  OutScaling=2^0  OutDataTypeStr=uint8
  PIDL : Constant  Value=hex2dec('0B')  OutDataTypeMode=uint8  OutDataType=fixdt(1, 16)  OutScaling=2^0  OutDataTypeStr=uint8
  Slave Address{,1..3} (4 alike) : Constant  Value=slvaddr  OutDataTypeMode=uint8  OutDataType=fixdt(1, 16)  OutScaling=2^0  OutDataTypeStr=uint8
  Terminator{,1..3} (4 alike) : Terminator
  Out1 : Outport
  wires:
  I2C Master Read/Write3/2 -> Terminator3/1
  I2C Master Read/Write2/2 -> Terminator2/1
  I2C Master Read/Write1/2 -> Terminator1/1
  I2C Master Read/Write/2 -> Terminator/1
  Logical Operator/1 -> Out1/1
  Compare To Zero2/1 -> Logical Operator/3
  Compare To Zero3/1 -> Logical Operator/4
  Compare To Zero1/1 -> Logical Operator/2
  Compare To Zero/1 -> Logical Operator/1
  I2C Master Read/Write3/1 -> Compare To Zero3/1
  I2C Master Read/Write2/1 -> Compare To Zero2/1
  I2C Master Read/Write1/1 -> Compare To Zero1/1
  I2C Master Read/Write/1 -> Compare To Zero/1
  PIDL/1 -> I2C Master Read/Write3/2
  Slave Address3/1 -> I2C Master Read/Write3/1
  PIDH/1 -> I2C Master Read/Write2/2
  Slave Address2/1 -> I2C Master Read/Write2/1
  MIDL/1 -> I2C Master Read/Write1/2
  Slave Address1/1 -> I2C Master Read/Write1/1
  MIDH/1 -> I2C Master Read/Write/2
  Slave Address/1 -> I2C Master Read/Write/1

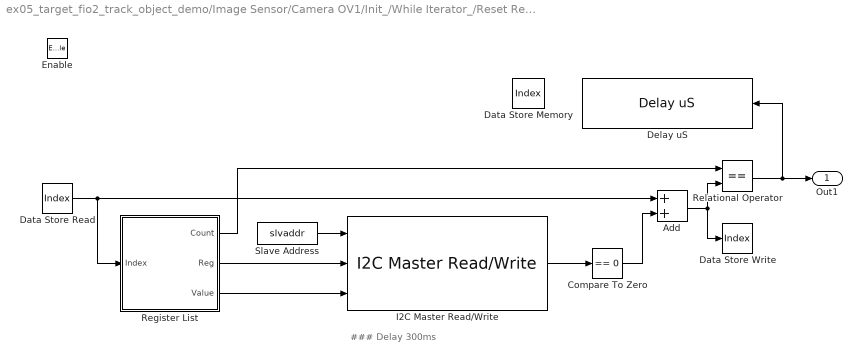
== system ex05_target_fio2_track_object_demo/Image Sensor/Camera OV1/Init_/While Iterator_/Reset Register_/Subsystem ==
  note: ### Delay 300ms
  Enable : EnablePort
  Add : Sum  OutDataType=fixdt(1, 16)  OutScaling=2^-10
  Compare To Zero : simulink/Logic and Bit Operations/Compare To Zero  SystemSampleTime=-1  relop===  LogicOutDataTypeMode=uint8  ZeroCross=off
  Data Store Memory : DataStoreMemory  DataStoreName=Index  ReadBeforeWriteMsg=warning  WriteAfterWriteMsg=warning  WriteAfterReadMsg=warning  DataType=uint8  OutDataType=fixdt(1, 16)  OutScaling=2^0  OutDataTypeStr=uint8
  Data Store Read : DataStoreRead  DataStoreName=Index  SampleTime=-1
  Data Store Write : DataStoreWrite  DataStoreName=Index  SampleTime=-1
  Delay uS : stm32f4_tim_lib/Delay uS  delaytime=200000  enableinput=on  enableoutput=off  inputtypearray=[1 -1]  outputtypearray=[0]  sampletime=-1  sampletimestr=0  blockid=ImageSensorCameraOV1Init_WhileIterator_ResetRegister_SubsystemDelayuS
  I2C Master Read/Write : stm32f4_i2c_lib/I2C Master Read//Write  configuration=Transaction  module=1  lastmodule=3  transfer=Blocking  dutycycle=TLow/THigh = 2  clkspeed=400  timeout=25  writecount=2  readcount=0  sdapin=C9  sclpin=A8  waitwritetime=300  forcestop=off  inputtypearray=[3 3 3 3]  outputtypearray=[1 3]  confstr="[\"C\",\"9\",\"A\",\"8\",\"1\",\"1\",\"6\",\"0\",\"I2C_DutyCycle_2\",\"300\",\"off\"]"  sampletime=-1  sampletimestr=0  blockid=ImageSensorCameraOV1Init_WhileIterator_ResetRegister_SubsystemI2CMasterReadWrite
  Register List : Subsystem  mask{register=uint8([hex2dec('12')]), value=uint8([hex2dec('80')])}
      mask prompts: register "Register Index"; value "Register Value"
      mask help:
      | Count:
      |  - Number of Register-Value pair.
      |  - Determine from lowest size, between Register and Value.
      | Reg:
      |  - Register index.
      | Value:
      |  - Data corresponding to specified register index.
  Relational Operator : RelationalOperator  Operator===  LogicOutDataTypeMode=boolean  LogicDataType=fixdt(0, 8)  OutDataTypeStr=boolean
  Slave Address : Constant  Value=slvaddr  OutDataTypeMode=uint8  OutDataType=fixdt(1, 16)  OutScaling=2^0  OutDataTypeStr=uint8
  Out1 : Outport
  wires:
  Slave Address/1 -> I2C Master Read/Write/1
  Data Store Read/1 -> Add/1, Register List/1(Index)
  I2C Master Read/Write/1 -> Compare To Zero/1
  Compare To Zero/1 -> Add/2
  Add/1 -> Relational Operator/2, Data Store Write/1
  Relational Operator/1 -> Delay uS/1, Out1/1
  Register List/2(Reg) -> I2C Master Read/Write/2
  Register List/3(Value) -> I2C Master Read/Write/3
  Register List/1(Count) -> Relational Operator/1

== system ex05_target_fio2_track_object_demo/Image Sensor/Camera OV1/Init_/While Iterator_/Clock Conf_/Subsystem/CLK24MHz_ ==
  Index : Inport  OutDataType=fixdt(1, 16)  OutScaling=2^0
  Enable : EnablePort
  Reg List_ : Subsystem  mask{register=uint8([17 107]), value=uint8([1 74])}
      mask prompts: register "Register Index"; value "Register Value"
      mask help:
      | Count:
      |  - Number of Register-Value pair.
      |  - Determine from lowest size, between Register and Value.
      | Reg:
      |  - Register index.
      | Value:
      |  - Data corresponding to specified register index.
  Count : Outport  OutDataType=fixdt(1, 16)  OutScaling=2^0
  Reg : Outport  Port=2  OutDataType=fixdt(1, 16)  OutScaling=2^0
  Value : Outport  Port=3  OutDataType=fixdt(1, 16)  OutScaling=2^0
  wires:
  Reg List_/1(Count) -> Count/1
  Reg List_/2(Reg) -> Reg/1
  Reg List_/3(Value) -> Value/1
  Index/1 -> Reg List_/1(Index)

== system ex05_target_fio2_track_object_demo/Image Sensor/Camera OV1/Init_/While Iterator_/Clock Conf_/Subsystem/CLK8MHz_ ==
  Index : Inport  OutDataType=fixdt(1, 16)  OutScaling=2^0
  Enable : EnablePort
  Reg List_ : Subsystem  mask{register=uint8([hex2dec('11') hex2dec('6B')]), value=uint8([hex2dec('00') hex2dec('80')])}
      mask prompts: register "Register Index"; value "Register Value"
      mask help:
      | Count:
      |  - Number of Register-Value pair.
      |  - Determine from lowest size, between Register and Value.
      | Reg:
      |  - Register index.
      | Value:
      |  - Data corresponding to specified register index.
  Count : Outport  OutDataType=fixdt(1, 16)  OutScaling=2^0
  Reg : Outport  Port=2  OutDataType=fixdt(1, 16)  OutScaling=2^0
  Value : Outport  Port=3  OutDataType=fixdt(1, 16)  OutScaling=2^0
  wires:
  Index/1 -> Reg List_/1(Index)
  Reg List_/3(Value) -> Value/1
  Reg List_/2(Reg) -> Reg/1
  Reg List_/1(Count) -> Count/1

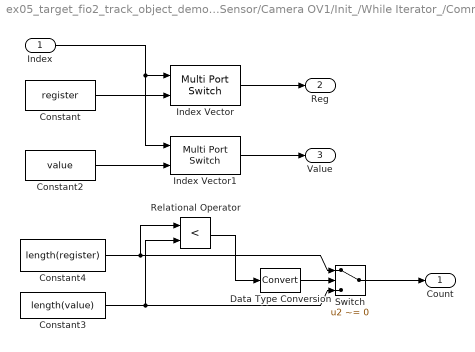
== system ex05_target_fio2_track_object_demo/Image Sensor/Camera OV1/Init_/While Iterator_/Common Conf_/Subsystem/Register List ==
  Index : Inport  OutDataType=fixdt(1, 16)  OutScaling=2^0
  Constant : Constant  Value=register  OutDataType=fixdt(1, 16)  OutScaling=2^0
  Constant2 : Constant  Value=value  OutDataType=fixdt(1, 16)  OutScaling=2^0
  Constant3 : Constant  Value=length(value)  OutDataType=fixdt(1, 16)  OutScaling=2^0
  Constant4 : Constant  Value=length(register)  OutDataType=fixdt(1, 16)  OutScaling=2^0
  Data Type Conversion : DataTypeConversion  OutDataType=fixdt(1, 16)  OutScaling=2^0
  Index Vector : MultiPortSwitch  Inputs=1  zeroidx=on  OutDataType=fixdt(1, 16)  OutScaling=2^0
  Index Vector1 : MultiPortSwitch  Inputs=1  zeroidx=on  OutDataType=fixdt(1, 16)  OutScaling=2^0
  Relational Operator : RelationalOperator  Operator=<  LogicOutDataTypeMode=boolean  LogicDataType=fixdt(0, 8)  OutDataTypeStr=boolean
  Switch : Switch  Criteria=u2 ~= 0  OutDataType=fixdt(1, 16)  OutScaling=2^0
  Count : Outport  OutDataType=fixdt(1, 16)  OutScaling=2^0
  Reg : Outport  Port=2  OutDataType=fixdt(1, 16)  OutScaling=2^0
  Value : Outport  Port=3  OutDataType=fixdt(1, 16)  OutScaling=2^0
  wires:
  Data Type Conversion/1 -> Switch/2
  Switch/1 -> Count/1
  Relational Operator/1 -> Data Type Conversion/1
  Constant3/1 -> Switch/3, Relational Operator/2
  Constant4/1 -> Switch/1, Relational Operator/1
  Index Vector1/1 -> Value/1
  Constant2/1 -> Index Vector1/2
  Index/1 -> Index Vector1/1, Index Vector/1
  Constant/1 -> Index Vector/2
  Index Vector/1 -> Reg/1

== system ex05_target_fio2_track_object_demo/Image Sensor/Camera OV1/Init_/While Iterator_/Picture Size_/Subsystem/Subsystem ==
  Index : Inport
  Constant : Constant  Value=imgsize  OutDataType=fixdt(1, 16)  OutScaling=2^0
  Img120x160 : Subsystem  TreatAsAtomicUnit=on
  Img240x320 : Subsystem  TreatAsAtomicUnit=on
  Img480x640 : Subsystem  TreatAsAtomicUnit=on
  Merge_Count : Merge  Inputs=3
  Merge_Reg : Merge  Inputs=3
  Merge_Value : Merge  Inputs=3
  Switch Case : SwitchCase  CaseConditions={1,2}
  Count : Outport
  Reg : Outport  Port=2
  Value : Outport  Port=3
  wires:
  Switch Case/3 -> Img480x640/Action
  Constant/1 -> Switch Case/1
  Merge_Value/1 -> Value/1
  Merge_Reg/1 -> Reg/1
  Merge_Count/1 -> Count/1
  Index/1 -> Img480x640/1(Index), Img240x320/1(Index), Img120x160/1(Index)
  Img480x640/3(Value) -> Merge_Value/3
  Img240x320/3(Value) -> Merge_Value/2
  Img120x160/3(Value) -> Merge_Value/1
  Img480x640/2(Reg) -> Merge_Reg/3
  Img240x320/2(Reg) -> Merge_Reg/2
  Img120x160/2(Reg) -> Merge_Reg/1
  Img240x320/1(Count) -> Merge_Count/2
  Img480x640/1(Count) -> Merge_Count/3
  Img120x160/1(Count) -> Merge_Count/1
  Switch Case/2 -> Img240x320/Action
  Switch Case/1 -> Img120x160/Action

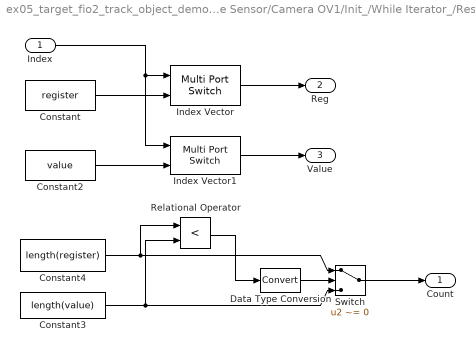
== system ex05_target_fio2_track_object_demo/Image Sensor/Camera OV1/Init_/While Iterator_/Reset Register_/Subsystem/Register List ==
  Index : Inport  OutDataType=fixdt(1, 16)  OutScaling=2^0
  Constant : Constant  Value=register  OutDataType=fixdt(1, 16)  OutScaling=2^0
  Constant2 : Constant  Value=value  OutDataType=fixdt(1, 16)  OutScaling=2^0
  Constant3 : Constant  Value=length(value)  OutDataType=fixdt(1, 16)  OutScaling=2^0
  Constant4 : Constant  Value=length(register)  OutDataType=fixdt(1, 16)  OutScaling=2^0
  Data Type Conversion : DataTypeConversion  OutDataType=fixdt(1, 16)  OutScaling=2^0
  Index Vector : MultiPortSwitch  Inputs=1  zeroidx=on  OutDataType=fixdt(1, 16)  OutScaling=2^0
  Index Vector1 : MultiPortSwitch  Inputs=1  zeroidx=on  OutDataType=fixdt(1, 16)  OutScaling=2^0
  Relational Operator : RelationalOperator  Operator=<  LogicOutDataTypeMode=boolean  LogicDataType=fixdt(0, 8)  OutDataTypeStr=boolean
  Switch : Switch  Criteria=u2 ~= 0  OutDataType=fixdt(1, 16)  OutScaling=2^0
  Count : Outport  OutDataType=fixdt(1, 16)  OutScaling=2^0
  Reg : Outport  Port=2  OutDataType=fixdt(1, 16)  OutScaling=2^0
  Value : Outport  Port=3  OutDataType=fixdt(1, 16)  OutScaling=2^0
  wires:
  Data Type Conversion/1 -> Switch/2
  Switch/1 -> Count/1
  Relational Operator/1 -> Data Type Conversion/1
  Constant3/1 -> Switch/3, Relational Operator/2
  Constant4/1 -> Switch/1, Relational Operator/1
  Index Vector1/1 -> Value/1
  Constant2/1 -> Index Vector1/2
  Index/1 -> Index Vector1/1, Index Vector/1
  Constant/1 -> Index Vector/2
  Index Vector/1 -> Reg/1

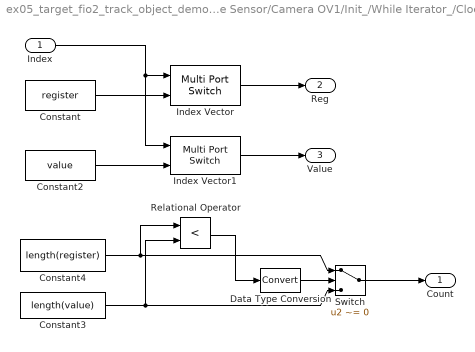
== system ex05_target_fio2_track_object_demo/Image Sensor/Camera OV1/Init_/While Iterator_/Clock Conf_/Subsystem/CLK24MHz_/Reg List_ ==
  Index : Inport  OutDataType=fixdt(1, 16)  OutScaling=2^0
  Constant : Constant  Value=register  OutDataType=fixdt(1, 16)  OutScaling=2^0
  Constant2 : Constant  Value=value  OutDataType=fixdt(1, 16)  OutScaling=2^0
  Constant3 : Constant  Value=length(value)  OutDataType=fixdt(1, 16)  OutScaling=2^0
  Constant4 : Constant  Value=length(register)  OutDataType=fixdt(1, 16)  OutScaling=2^0
  Data Type Conversion : DataTypeConversion  OutDataType=fixdt(1, 16)  OutScaling=2^0
  Index Vector : MultiPortSwitch  Inputs=1  zeroidx=on  OutDataType=fixdt(1, 16)  OutScaling=2^0
  Index Vector1 : MultiPortSwitch  Inputs=1  zeroidx=on  OutDataType=fixdt(1, 16)  OutScaling=2^0
  Relational Operator : RelationalOperator  Operator=<  LogicOutDataTypeMode=boolean  LogicDataType=fixdt(0, 8)  OutDataTypeStr=boolean
  Switch : Switch  Criteria=u2 ~= 0  OutDataType=fixdt(1, 16)  OutScaling=2^0
  Count : Outport  OutDataType=fixdt(1, 16)  OutScaling=2^0
  Reg : Outport  Port=2  OutDataType=fixdt(1, 16)  OutScaling=2^0
  Value : Outport  Port=3  OutDataType=fixdt(1, 16)  OutScaling=2^0
  wires:
  Data Type Conversion/1 -> Switch/2
  Switch/1 -> Count/1
  Relational Operator/1 -> Data Type Conversion/1
  Constant3/1 -> Switch/3, Relational Operator/2
  Constant4/1 -> Switch/1, Relational Operator/1
  Index Vector1/1 -> Value/1
  Constant2/1 -> Index Vector1/2
  Index/1 -> Index Vector1/1, Index Vector/1
  Constant/1 -> Index Vector/2
  Index Vector/1 -> Reg/1

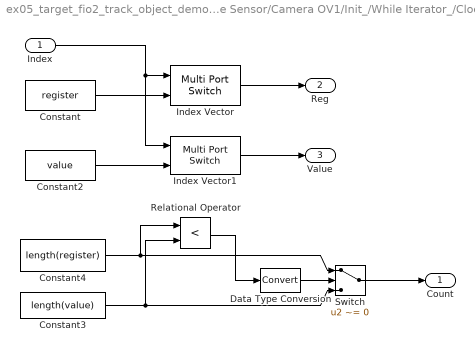
== system ex05_target_fio2_track_object_demo/Image Sensor/Camera OV1/Init_/While Iterator_/Clock Conf_/Subsystem/CLK8MHz_/Reg List_ ==
  Index : Inport  OutDataType=fixdt(1, 16)  OutScaling=2^0
  Constant : Constant  Value=register  OutDataType=fixdt(1, 16)  OutScaling=2^0
  Constant2 : Constant  Value=value  OutDataType=fixdt(1, 16)  OutScaling=2^0
  Constant3 : Constant  Value=length(value)  OutDataType=fixdt(1, 16)  OutScaling=2^0
  Constant4 : Constant  Value=length(register)  OutDataType=fixdt(1, 16)  OutScaling=2^0
  Data Type Conversion : DataTypeConversion  OutDataType=fixdt(1, 16)  OutScaling=2^0
  Index Vector : MultiPortSwitch  Inputs=1  zeroidx=on  OutDataType=fixdt(1, 16)  OutScaling=2^0
  Index Vector1 : MultiPortSwitch  Inputs=1  zeroidx=on  OutDataType=fixdt(1, 16)  OutScaling=2^0
  Relational Operator : RelationalOperator  Operator=<  LogicOutDataTypeMode=boolean  LogicDataType=fixdt(0, 8)  OutDataTypeStr=boolean
  Switch : Switch  Criteria=u2 ~= 0  OutDataType=fixdt(1, 16)  OutScaling=2^0
  Count : Outport  OutDataType=fixdt(1, 16)  OutScaling=2^0
  Reg : Outport  Port=2  OutDataType=fixdt(1, 16)  OutScaling=2^0
  Value : Outport  Port=3  OutDataType=fixdt(1, 16)  OutScaling=2^0
  wires:
  Index Vector/1 -> Reg/1
  Constant/1 -> Index Vector/2
  Index/1 -> Index Vector/1, Index Vector1/1
  Constant2/1 -> Index Vector1/2
  Index Vector1/1 -> Value/1
  Constant4/1 -> Relational Operator/1, Switch/1
  Constant3/1 -> Relational Operator/2, Switch/3
  Relational Operator/1 -> Data Type Conversion/1
  Switch/1 -> Count/1
  Data Type Conversion/1 -> Switch/2

== system ex05_target_fio2_track_object_demo/Image Sensor/Camera OV1/Init_/While Iterator_/Picture Size_/Subsystem/Subsystem/Img120x160 ==
  Index : Inport  OutDataType=fixdt(1, 16)  OutScaling=2^0
  Action Port : ActionPort  ActionType=case
  Register List : Subsystem  mask{register=uint8([58,61,140,64,18,50,23,24,25,26,3,12,62,112,113,114,115,162]), value=uint8([8,192,0,208,20,128,22,4,3,123,10,4,26,58,53,238,242,2])}
      mask prompts: register "Register Index"; value "Register Value"
      mask help:
      | Count:
      |  - Number of Register-Value pair.
      |  - Determine from lowest size, between Register and Value.
      | Reg:
      |  - Register index.
      | Value:
      |  - Data corresponding to specified register index.
  Count : Outport  OutDataType=fixdt(1, 16)  OutScaling=2^0
  Reg : Outport  Port=2  OutDataType=fixdt(1, 16)  OutScaling=2^0
  Value : Outport  Port=3  OutDataType=fixdt(1, 16)  OutScaling=2^0
  wires:
  Register List/3(Value) -> Value/1
  Register List/2(Reg) -> Reg/1
  Register List/1(Count) -> Count/1
  Index/1 -> Register List/1(Index)

== system ex05_target_fio2_track_object_demo/Image Sensor/Camera OV1/Init_/While Iterator_/Picture Size_/Subsystem/Subsystem/Img240x320 ==
  Index : Inport  OutDataType=fixdt(1, 16)  OutScaling=2^0
  Action Port : ActionPort  ActionType=case
  Register List : Subsystem  mask{register=uint8([58,61,140,64,18,50,23,24,25,26,3,12,62,112,113,114,115,162]), value=uint8([8,130,0,208,20,128,22,4,3,123,10,4,0,58,53,17,240,2])}
      mask prompts: register "Register Index"; value "Register Value"
      mask help:
      | Count:
      |  - Number of Register-Value pair.
      |  - Determine from lowest size, between Register and Value.
      | Reg:
      |  - Register index.
      | Value:
      |  - Data corresponding to specified register index.
  Count : Outport  OutDataType=fixdt(1, 16)  OutScaling=2^0
  Reg : Outport  Port=2  OutDataType=fixdt(1, 16)  OutScaling=2^0
  Value : Outport  Port=3  OutDataType=fixdt(1, 16)  OutScaling=2^0
  wires:
  Index/1 -> Register List/1(Index)
  Register List/1(Count) -> Count/1
  Register List/2(Reg) -> Reg/1
  Register List/3(Value) -> Value/1
